simulink model "ECS_FOS"  (Simulink 8.2)
settings: Solver=ode45  StartTime=0.0  StopTime=18000  RelTol=1e-3
InitFcn:
  | load('loss_coeff_mixing_junction.mat')
  | load('SampleOutput.mat')
  | load('HydProp.mat')
  | load('HydraulicLoad.mat')
  | load('initavload.mat')
  | load('SampleFuelBurn.mat')
values from neighbouring files (symbols this model uses):
  FuelBurn = [0 0 0 0 0 0 0 0 0 0 0 0 ... (18249 elements, 1x18249)]    [Benchmark_data1.mat]
  fueltankdata =     [Benchmark_data1.mat]
undefined symbols (not defined in the file or in its folder): AirProp, F1, F2, HUGHES_TREITLER, magnitude, PN_70147, PumpProp
libraries: PowerFlowLib x46, simulink x4
(part 4 of 5)

== system ECS_FOS/ECS/Fuel Tanks/Pumps/Fuel Control Right Wing  ==
  FuelNeed : Inport
  FuelFromPump : Inport  Port=2
  Bus Creator : BusCreator  Inputs=3
  Bus Creator1 : BusCreator  Inputs=3
  Bus Selector : BusSelector  OutputSignals=mdot_kgps,temp_K,pres_kPa
  Gain : Gain
  Gain1 : Gain
  Saturation : Saturate  UpperLimit=inf  LowerLimit=0
  Sum : Sum  Inputs=|+-
  Switch : Switch  Criteria=u2 > Threshold
  Fuel2Engine : Outport
  Fuel2Tank : Outport  Port=2
  wires:
  Gain1/1 -> Bus Creator1/2  "temp_K"
  Gain/1 -> Bus Creator1/3  "pres_kPa"
  Bus Creator1/1 -> Fuel2Engine/1
  Bus Selector/3 -> Gain/1, Bus Creator/3  "<pres_kPa>"
  Switch/1 -> Bus Creator1/1  "mdot_kgps"
  Saturation/1 -> Bus Creator/1  "mdot_kgps"
  Bus Selector/2 -> Gain1/1, Bus Creator/2  "<temp_K>"
  Bus Creator/1 -> Fuel2Tank/1
  Sum/1 -> Switch/2, Saturation/1
  FuelNeed/1 -> Switch/1, Sum/2
  Bus Selector/1 -> Switch/3, Sum/1  "<mdot_kgps>"
  FuelFromPump/1 -> Bus Selector/1

== system ECS_FOS/ECS/Fuel Tanks/Pumps/Fuel Switch On/Off ==
  Right Wing Tank : Inport
  Center Tank : Inport  Port=2
  Left Wing Tank : Inport  Port=3
  Operating RPM : Constant  Value=6000
  Operating RPM1 : Constant  Value=6000
  Operating RPM2 : Constant  Value=6000
  Right Wing Fuel  Pumps On/Off : Switch  Criteria=u2 ~= 0
  Right Wing Fuel  Pumps On/Off1 : Switch  Criteria=u2 ~= 0
  Right Wing Fuel  Pumps On/Off2 : Switch  Criteria=u2 ~= 0
  shut off : Constant  Value=0
  shut off1 : Constant  Value=0
  shut off2 : Constant  Value=0
  Right Wing RPM : Outport
  Left Wing RPM : Outport  Port=2
  Center RPM : Outport  Port=3
  wires:
  Right Wing Fuel  Pumps On/Off2/1 -> Left Wing RPM/1
  Right Wing Fuel  Pumps On/Off1/1 -> Center RPM/1
  Right Wing Fuel  Pumps On/Off/1 -> Right Wing RPM/1
  Left Wing Tank/1 -> Right Wing Fuel  Pumps On/Off2/2
  shut off2/1 -> Right Wing Fuel  Pumps On/Off2/3
  Operating RPM2/1 -> Right Wing Fuel  Pumps On/Off2/1
  Center Tank/1 -> Right Wing Fuel  Pumps On/Off1/2
  shut off1/1 -> Right Wing Fuel  Pumps On/Off1/3
  Operating RPM1/1 -> Right Wing Fuel  Pumps On/Off1/1
  Right Wing Tank/1 -> Right Wing Fuel  Pumps On/Off/2
  shut off/1 -> Right Wing Fuel  Pumps On/Off/3
  Operating RPM/1 -> Right Wing Fuel  Pumps On/Off/1

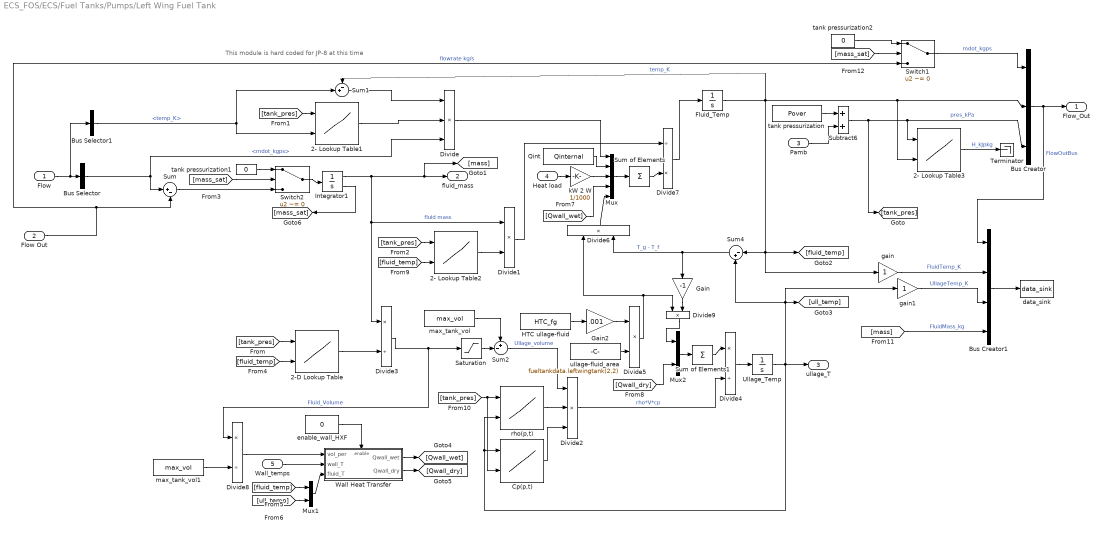
== system ECS_FOS/ECS/Fuel Tanks/Pumps/Left Wing Fuel Tank ==
  note: This module is hard coded for JP-8 at this time
  Flow : Inport
  Flow Out : Inport  Port=2
  Pamb : Inport  Port=3
  Heat load : Inport  Port=4
  Wall_temps : Inport  Port=5
  2- Lookup Table1 : Lookup_n-D  BreakpointsForDimension1=F1.P  BreakpointsForDimension2=F1.T  Table=F1.Cp_pt  RndMeth=Simplest  InputSameDT=on
  2- Lookup Table2 : Lookup_n-D  BreakpointsForDimension1=F1.P  BreakpointsForDimension2=F1.T  Table=F1.Cp_pt  RndMeth=Simplest  InputSameDT=on
  2- Lookup Table3 : Lookup_n-D  BreakpointsForDimension1=F1.P  BreakpointsForDimension2=F1.T  Table=F1.H_pt  RndMeth=Simplest  InputSameDT=on
  2-D Lookup Table : Lookup_n-D  BreakpointsForDimension1=F1.P  BreakpointsForDimension2=F1.T  Table=F1.Rho_pt  RndMeth=Simplest  InputSameDT=on
  Bus Creator : BusCreator  Inputs=3
  Bus Creator1 : BusCreator
  Bus Selector : BusSelector  OutputSignals=mdot_kgps
  Bus Selector1 : BusSelector  OutputSignals=temp_K
  Cp(p,t) : Lookup_n-D  BreakpointsForDimension1=AirProp.P  BreakpointsForDimension2=AirProp.T  Table=AirProp.Cp_pt  RndMeth=Simplest  InputSameDT=on
  Divide : Product  Inputs=***
  Divide{1,5..6,9} (4 alike) : Product  Inputs=**
  Divide2 : Product  Inputs=***
  Divide3 : Product  Inputs=*/
  Divide4 : Product  Inputs=*/
  Divide7 : Product  Inputs=/*
  Divide8 : Product  Inputs=*/
  Fluid_Temp : Integrator  InitialCondition=fld_Tint + 273.15  LimitOutput=on  UpperSaturationLimit=800  LowerSaturationLimit=eps
  Gain : Gain  Gain=-1
  Gain2 : Gain  Gain=.001
  HTC ullage-fluid : Constant  Value=HTC_fg
  Integrator1 : Integrator  InitialCondition=m_init  LimitOutput=on  LowerSaturationLimit=1  ShowSaturationPort=on
  Mux : Mux  Inputs=5
  Mux1 : Mux  Inputs=2
  Mux2 : Mux  Inputs=2
  Qint : Constant  Value=Qinternal
  Saturation : Saturate  UpperLimit=inf  LowerLimit=eps  ZeroCross=off
  Subtract6 : Sum
  Sum : Sum  Inputs=|+-
  Sum of Elements : Sum  Inputs=+
  Sum of Elements1 : Sum  Inputs=+
  Sum1 : Sum  Inputs=-+|
  Sum2 : Sum  Inputs=+-|
  Sum4 : Sum  Inputs=|-+
  Switch1 : Switch  Criteria=u2 ~= 0  Threshold=-1
  Switch2 : Switch  Criteria=u2 ~= 0  Threshold=-1
  Terminator : Terminator
  Ullage_Temp : Integrator  InitialCondition=ull_Tint + 273.15  LimitOutput=on  LowerSaturationLimit=eps
  Wall Heat Transfer : Subsystem  TreatAsAtomicUnit=on
  data_sink : PowerFlowLib/Support Functions//Tools/data_sink
      link override global_data_goto: GotoTag=gdata_PowerFlowLibEnergyPowerSystemsThermalFuelFuelTank
  enable_wall_HXF : Constant  Value=0
  gain : Gain
  gain1 : Gain
  kW 2 W : Gain  Gain=1/1000
  max_tank_vol : Constant  Value=max_vol
  max_tank_vol1 : Constant  Value=max_vol
  rho(p,t) : Lookup_n-D  BreakpointsForDimension1=AirProp.P  BreakpointsForDimension2=AirProp.T  Table=AirProp.Rho_pt  RndMeth=Simplest  InputSameDT=on
  tank pressurization : Constant  Value=Pover
  tank pressurization1 : Constant  Value=0
  tank pressurization2 : Constant  Value=0
  ullage-fluid_area : Constant  Value=fueltankdata.leftwingtank(2,2)
  Flow_Out : Outport
  fluid_mass : Outport  Port=2
  ullage_T : Outport  Port=3
  wires:
  Switch2/1 -> Integrator1/1
  tank pressurization1/1 -> Switch2/1
  [mass_sat] -> Switch2/2
  Integrator1/2 -> [mass_sat]
  Sum/1 -> Switch2/3
  tank pressurization2/1 -> Switch1/1
  [mass_sat] -> Switch1/2
  [mass] -> Bus Creator1/4  "FluidMass_kg"
  gain1/1 -> Bus Creator1/3  "UllageTemp_K"
  gain/1 -> Bus Creator1/2  "FluidTemp_K"
  Bus Creator1/1 -> data_sink/1
  kW 2 W/1 -> Mux/3
  2- Lookup Table3/1 -> Terminator/1  "H_kJpkg"
  Flow/1 -> Bus Selector/1, Bus Selector1/1
  Bus Selector/1 -> Divide/3, Sum/1  "<mdot_kgps>"
  Flow Out/1 -> Sum/2, Switch1/3  "flowrate kg/s"
  Integrator1/1 -> fluid_mass/1, [mass], Divide3/1, Divide1/1  "fluid mass"
  Bus Selector1/1 -> Sum1/2, 2- Lookup Table1/2  "<temp_K>"
  Sum1/1 -> Divide/1
  2- Lookup Table2/1 -> Divide1/2
  rho(p,t)/1 -> Divide2/2
  Cp(p,t)/1 -> Divide2/3
  Divide3/1 -> Saturation/1, Divide8/1  "Fluid_Volume"
  max_tank_vol/1 -> Sum2/1
  Sum2/1 -> Divide2/1  "Ullage_volume"
  Divide4/1 -> Ullage_Temp/1
  Ullage_Temp/1 -> ullage_T/1, gain1/1, Sum4/2, [ull_temp], rho(p,t)/2, Cp(p,t)/1
  Fluid_Temp/1 -> 2- Lookup Table3/2, Bus Creator/2, Sum1/1, gain/1, Sum4/1, [fluid_temp]  "temp_K"
  HTC ullage-fluid/1 -> Gain2/1
  ullage-fluid_area/1 -> Divide5/2
  Sum4/1 -> Divide6/2, Gain/1  "T_g - T_f"
  Divide1/1 -> Divide7/1
  Divide7/1 -> Fluid_Temp/1
  Divide5/1 -> Divide6/1, Divide9/1
  Pamb/1 -> Subtract6/2
  tank pressurization/1 -> Subtract6/1
  Subtract6/1 -> 2- Lookup Table3/1, Bus Creator/3, [tank_pres]  "pres_kPa"
  Bus Creator/1 -> Bus Creator1/1, Flow_Out/1  "FlowOutBus"
  Saturation/1 -> Sum2/2
  [tank_pres] -> 2-D Lookup Table/1
  2-D Lookup Table/1 -> Divide3/2
  [tank_pres] -> 2- Lookup Table1/1
  2- Lookup Table1/1 -> Divide/2
  [tank_pres] -> 2- Lookup Table2/1
  max_tank_vol1/1 -> Divide8/2
  Switch1/1 -> Bus Creator/1  "mdot_kgps"
  Divide/1 -> Mux/1
  Qint/1 -> Mux/2
  Heat load/1 -> kW 2 W/1
  Sum of Elements/1 -> Divide7/2
  Mux/1 -> Sum of Elements/1
  [fluid_temp] -> 2-D Lookup Table/2
  Divide8/1 -> Wall Heat Transfer/1(vol_per)
  Wall_temps/1 -> Wall Heat Transfer/2(wall_T)
  [fluid_temp] -> Mux1/1
  [ull_temp] -> Mux1/2
  Mux1/1 -> Wall Heat Transfer/3(fluid_T)
  Wall Heat Transfer/1(Qwall_wet) -> [Qwall_wet]
  Wall Heat Transfer/2(Qwall_dry) -> [Qwall_dry]
  Divide6/1 -> Mux/5
  Divide2/1 -> Divide4/2  "rho*V*cp"
  Mux2/1 -> Sum of Elements1/1
  Sum of Elements1/1 -> Divide4/1
  Gain/1 -> Divide9/2
  Divide9/1 -> Mux2/1
  [Qwall_dry] -> Mux2/2
  [Qwall_wet] -> Mux/4
  [fluid_temp] -> 2- Lookup Table2/2
  enable_wall_HXF/1 -> Wall Heat Transfer/Enable
  Gain2/1 -> Divide5/1
  [tank_pres] -> rho(p,t)/1, Cp(p,t)/2

== system ECS_FOS/ECS/Fuel Tanks/Pumps/Pump Split1 ==
  Flow In : Inport
  Bus Creator : BusCreator  Inputs=3
  Bus Selector14 : BusSelector  OutputSignals=temp_K,mdot_kgps,pres_kPa
  Gain : Gain  Gain=0.5
  Flow Out : Outport
  wires:
  Bus Selector14/3 -> Bus Creator/3  "<pres_kPa>"
  Gain/1 -> Bus Creator/2  "mdot_kgps"
  Bus Selector14/1 -> Bus Creator/1  "<temp_K>"
  Bus Creator/1 -> Flow Out/1
  Bus Selector14/2 -> Gain/1  "<mdot_kgps>"
  Flow In/1 -> Bus Selector14/1

== system ECS_FOS/ECS/Fuel Tanks/Pumps/Pump Split2 ==
  Flow In : Inport
  Bus Creator : BusCreator  Inputs=3
  Bus Selector14 : BusSelector  OutputSignals=temp_K,mdot_kgps,pres_kPa
  Gain : Gain  Gain=0.5
  Flow Out : Outport
  wires:
  Flow In/1 -> Bus Selector14/1
  Bus Selector14/2 -> Gain/1  "<mdot_kgps>"
  Bus Creator/1 -> Flow Out/1
  Bus Selector14/1 -> Bus Creator/1  "<temp_K>"
  Gain/1 -> Bus Creator/2  "mdot_kgps"
  Bus Selector14/3 -> Bus Creator/3  "<pres_kPa>"

== system ECS_FOS/ECS/Fuel Tanks/Pumps/Pump Split3 ==
  Flow In : Inport
  Bus Creator : BusCreator  Inputs=3
  Bus Selector14 : BusSelector  OutputSignals=temp_K,mdot_kgps,pres_kPa
  Gain : Gain  Gain=0.5
  Flow Out : Outport
  wires:
  Bus Selector14/3 -> Bus Creator/3  "<pres_kPa>"
  Gain/1 -> Bus Creator/2  "mdot_kgps"
  Bus Selector14/1 -> Bus Creator/1  "<temp_K>"
  Bus Creator/1 -> Flow Out/1
  Bus Selector14/2 -> Gain/1  "<mdot_kgps>"
  Flow In/1 -> Bus Selector14/1

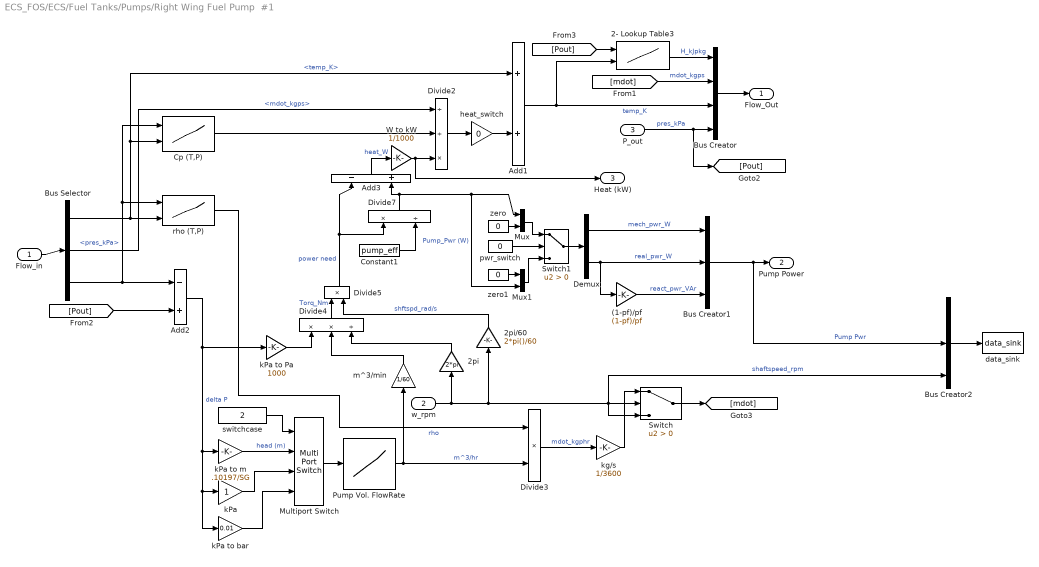
== system ECS_FOS/ECS/Fuel Tanks/Pumps/Right Wing Fuel Pump  #1 ==
  Flow_in : Inport
  w_rpm : Inport  Port=2
  P_out : Inport  Port=3
  (1-pf)/pf : Gain  Gain=(1-pf)/pf
  2- Lookup Table3 : Lookup_n-D  BreakpointsForDimension1=F1.P  BreakpointsForDimension2=F1.T  Table=F1.H_pt  RndMeth=Simplest  InputSameDT=on
  2pi : Gain  Gain=2*pi
  2pi/60 : Gain  Gain=2*pi()/60
  Add1 : Sum
  Add2 : Sum  Inputs=-+
  Add3 : Sum  Inputs=-+
  Bus Creator : BusCreator
  Bus Creator1 : BusCreator  Inputs=3
  Bus Creator2 : BusCreator  Inputs=3
  Bus Selector : BusSelector  OutputSignals=temp_K,mdot_kgps,pres_kPa
  Constant1 : Constant  Value=pump_eff
  Cp (T,P) : Lookup_n-D  BreakpointsForDimension1=F1.P  BreakpointsForDimension2=F1.T  Table=F1.Cp_pt  RndMeth=Simplest  InputSameDT=on
  Demux : Demux  Outputs=2
  Divide2 : Product  Inputs=//*
  Divide3 : Product  Inputs=**
  Divide4 : Product  Inputs=**/
  Divide5 : Product  Inputs=**
  Divide7 : Product  Inputs=*/
  Multiport Switch : MultiPortSwitch
  Mux : Mux  Inputs=2
  Mux1 : Mux  Inputs=2
  Pump Vol. FlowRate : Lookup_n-D  NumberOfTableDimensions=1  BreakpointsForDimension1=PumpProp.B737_AC_fuel1.pres  Table=PumpProp.B737_AC_fuel1.q  RndMeth=Simplest  InputSameDT=on
  Switch : Switch  Criteria=u2 > Threshold
  Switch1 : Switch  Criteria=u2 > Threshold
  W to kW : Gain  Gain=1/1000
  data_sink : PowerFlowLib/Support Functions//Tools/data_sink
  heat_switch : Gain  Gain=0
  "kPa " : Gain
  kPa to Pa : Gain  Gain=1000
  kPa to bar : Gain  Gain=0.01
  kPa to m : Gain  Gain=.10197/SG
  kg/s : Gain  Gain=1/3600
  m^3/min : Gain  Gain=1/60
  pwr_switch : Constant  Value=0
  rho (T,P) : Lookup_n-D  BreakpointsForDimension1=F1.P  BreakpointsForDimension2=F1.T  Table=F1.Rho_pt  RndMeth=Simplest  InputSameDT=on
  switchcase : Constant  Value=2
  zero : Constant  Value=0
  zero1 : Constant  Value=0
  Flow_Out : Outport
  Pump Power : Outport  Port=2
  Heat (kW) : Outport  Port=3
  wires:
  Bus Creator2/1 -> data_sink/1
  heat_switch/1 -> Add1/2
  Mux1/1 -> Switch1/3
  zero1/1 -> Mux1/1
  W to kW/1 -> Divide2/3, Heat (kW)/1
  zero/1 -> Mux/2
  Mux/1 -> Switch1/1
  pwr_switch/1 -> Switch1/2
  Switch1/1 -> Demux/1
  (1-pf)/pf/1 -> Bus Creator1/3  "react_pwr_VAr"
  Demux/2 -> (1-pf)/pf/1, Bus Creator1/2  "real_pwr_W"
  Bus Creator1/1 -> Bus Creator2/2, Pump Power/1  "Pump Pwr"
  Demux/1 -> Bus Creator1/1  "mech_pwr_W"
  Add3/1 -> W to kW/1  "heat_W"
  2pi/1 -> Divide4/3
  Divide7/1 -> Mux1/2, Mux/1, Add3/2  "Pump_Pwr (W)"
  m^3/min/1 -> Divide4/2
  kPa to Pa/1 -> Divide4/1
  Divide5/1 -> Add3/1, Divide7/1  "power need"
  2pi/60/1 -> Divide5/2  "shftspd_rad/s"
  Switch/1 -> [mdot]
  kg/s/1 -> Switch/1
  [Pout] -> 2- Lookup Table3/1
  P_out/1 -> Bus Creator/4, [Pout]  "pres_kPa"
  2- Lookup Table3/1 -> Bus Creator/1  "H_kJpkg"
  Flow_in/1 -> Bus Selector/1
  Bus Creator/1 -> Flow_Out/1
  Divide2/1 -> heat_switch/1
  Cp (T,P)/1 -> Divide2/2
  Constant1/1 -> Divide7/2
  Bus Selector/2 -> Divide2/1  "<mdot_kgps>"
  rho (T,P)/1 -> Divide3/1  "rho"
  Bus Selector/1 -> rho (T,P)/2, Add1/1, Cp (T,P)/2  "<temp_K>"
  Bus Selector/3 -> rho (T,P)/1, Cp (T,P)/1, Add2/1  "<pres_kPa>"
  Add2/1 -> kPa to Pa/1, kPa to m/1, "kPa "/1, kPa to bar/1  "delta P"
  Add1/1 -> 2- Lookup Table3/2, Bus Creator/3  "temp_K"
  w_rpm/1 -> Bus Creator2/3, Switch/3, Switch/2, 2pi/60/1, 2pi/1  "shaftspeed_rpm"
  [mdot] -> Bus Creator/2  "mdot_kgps"
  [Pout] -> Add2/2
  kPa to m/1 -> Multiport Switch/2  "head (m)"
  Divide3/1 -> kg/s/1  "mdot_kgphr"
  Pump Vol. FlowRate/1 -> Divide3/2, m^3/min/1  "m^3/hr"
  Divide4/1 -> Divide5/1  "Torq_Nm"
  switchcase/1 -> Multiport Switch/1
  Multiport Switch/1 -> Pump Vol. FlowRate/1
  "kPa "/1 -> Multiport Switch/3
  kPa to bar/1 -> Multiport Switch/4

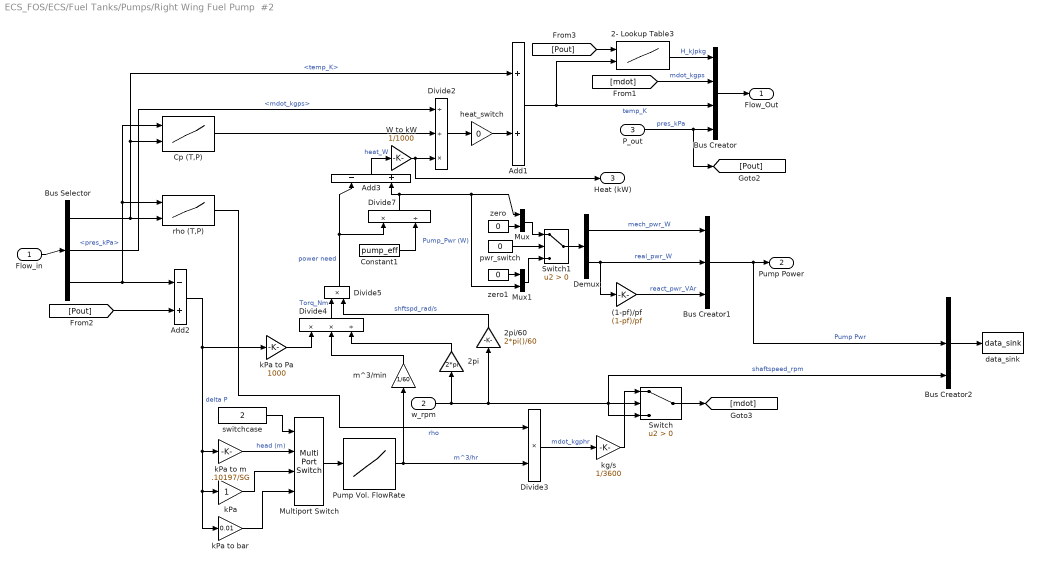
== system ECS_FOS/ECS/Fuel Tanks/Pumps/Right Wing Fuel Pump  #2 ==
  Flow_in : Inport
  w_rpm : Inport  Port=2
  P_out : Inport  Port=3
  (1-pf)/pf : Gain  Gain=(1-pf)/pf
  2- Lookup Table3 : Lookup_n-D  BreakpointsForDimension1=F1.P  BreakpointsForDimension2=F1.T  Table=F1.H_pt  RndMeth=Simplest  InputSameDT=on
  2pi : Gain  Gain=2*pi
  2pi/60 : Gain  Gain=2*pi()/60
  Add1 : Sum
  Add2 : Sum  Inputs=-+
  Add3 : Sum  Inputs=-+
  Bus Creator : BusCreator
  Bus Creator1 : BusCreator  Inputs=3
  Bus Creator2 : BusCreator  Inputs=3
  Bus Selector : BusSelector  OutputSignals=temp_K,mdot_kgps,pres_kPa
  Constant1 : Constant  Value=pump_eff
  Cp (T,P) : Lookup_n-D  BreakpointsForDimension1=F1.P  BreakpointsForDimension2=F1.T  Table=F1.Cp_pt  RndMeth=Simplest  InputSameDT=on
  Demux : Demux  Outputs=2
  Divide2 : Product  Inputs=//*
  Divide3 : Product  Inputs=**
  Divide4 : Product  Inputs=**/
  Divide5 : Product  Inputs=**
  Divide7 : Product  Inputs=*/
  Multiport Switch : MultiPortSwitch
  Mux : Mux  Inputs=2
  Mux1 : Mux  Inputs=2
  Pump Vol. FlowRate : Lookup_n-D  NumberOfTableDimensions=1  BreakpointsForDimension1=PumpProp.B737_AC_fuel1.pres  Table=PumpProp.B737_AC_fuel1.q  RndMeth=Simplest  InputSameDT=on
  Switch : Switch  Criteria=u2 > Threshold
  Switch1 : Switch  Criteria=u2 > Threshold
  W to kW : Gain  Gain=1/1000
  data_sink : PowerFlowLib/Support Functions//Tools/data_sink
  heat_switch : Gain  Gain=0
  "kPa " : Gain
  kPa to Pa : Gain  Gain=1000
  kPa to bar : Gain  Gain=0.01
  kPa to m : Gain  Gain=.10197/SG
  kg/s : Gain  Gain=1/3600
  m^3/min : Gain  Gain=1/60
  pwr_switch : Constant  Value=0
  rho (T,P) : Lookup_n-D  BreakpointsForDimension1=F1.P  BreakpointsForDimension2=F1.T  Table=F1.Rho_pt  RndMeth=Simplest  InputSameDT=on
  switchcase : Constant  Value=2
  zero : Constant  Value=0
  zero1 : Constant  Value=0
  Flow_Out : Outport
  Pump Power : Outport  Port=2
  Heat (kW) : Outport  Port=3
  wires:
  kPa to bar/1 -> Multiport Switch/4
  "kPa "/1 -> Multiport Switch/3
  Multiport Switch/1 -> Pump Vol. FlowRate/1
  switchcase/1 -> Multiport Switch/1
  Divide4/1 -> Divide5/1  "Torq_Nm"
  Pump Vol. FlowRate/1 -> m^3/min/1, Divide3/2  "m^3/hr"
  Divide3/1 -> kg/s/1  "mdot_kgphr"
  kPa to m/1 -> Multiport Switch/2  "head (m)"
  [Pout] -> Add2/2
  [mdot] -> Bus Creator/2  "mdot_kgps"
  w_rpm/1 -> 2pi/1, 2pi/60/1, Switch/2, Switch/3, Bus Creator2/3  "shaftspeed_rpm"
  Add1/1 -> Bus Creator/3, 2- Lookup Table3/2  "temp_K"
  Add2/1 -> kPa to bar/1, "kPa "/1, kPa to m/1, kPa to Pa/1  "delta P"
  Bus Selector/3 -> Add2/1, Cp (T,P)/1, rho (T,P)/1  "<pres_kPa>"
  Bus Selector/1 -> Cp (T,P)/2, Add1/1, rho (T,P)/2  "<temp_K>"
  rho (T,P)/1 -> Divide3/1  "rho"
  Bus Selector/2 -> Divide2/1  "<mdot_kgps>"
  Constant1/1 -> Divide7/2
  Cp (T,P)/1 -> Divide2/2
  Divide2/1 -> heat_switch/1
  Bus Creator/1 -> Flow_Out/1
  Flow_in/1 -> Bus Selector/1
  2- Lookup Table3/1 -> Bus Creator/1  "H_kJpkg"
  P_out/1 -> [Pout], Bus Creator/4  "pres_kPa"
  [Pout] -> 2- Lookup Table3/1
  kg/s/1 -> Switch/1
  Switch/1 -> [mdot]
  2pi/60/1 -> Divide5/2  "shftspd_rad/s"
  Divide5/1 -> Divide7/1, Add3/1  "power need"
  kPa to Pa/1 -> Divide4/1
  m^3/min/1 -> Divide4/2
  Divide7/1 -> Add3/2, Mux/1, Mux1/2  "Pump_Pwr (W)"
  2pi/1 -> Divide4/3
  Add3/1 -> W to kW/1  "heat_W"
  Demux/1 -> Bus Creator1/1  "mech_pwr_W"
  Bus Creator1/1 -> Pump Power/1, Bus Creator2/2  "Pump Pwr"
  Demux/2 -> Bus Creator1/2, (1-pf)/pf/1  "real_pwr_W"
  (1-pf)/pf/1 -> Bus Creator1/3  "react_pwr_VAr"
  Switch1/1 -> Demux/1
  pwr_switch/1 -> Switch1/2
  Mux/1 -> Switch1/1
  zero/1 -> Mux/2
  W to kW/1 -> Heat (kW)/1, Divide2/3
  zero1/1 -> Mux1/1
  Mux1/1 -> Switch1/3
  heat_switch/1 -> Add1/2
  Bus Creator2/1 -> data_sink/1

== system ECS_FOS/ECS/Fuel Tanks/Pumps/Right Wing Fuel Pump  #3 ==
  Flow_in : Inport
  w_rpm : Inport  Port=2
  P_out : Inport  Port=3
  (1-pf)/pf : Gain  Gain=(1-pf)/pf
  2- Lookup Table3 : Lookup_n-D  BreakpointsForDimension1=F1.P  BreakpointsForDimension2=F1.T  Table=F1.H_pt  RndMeth=Simplest  InputSameDT=on
  2pi : Gain  Gain=2*pi
  2pi/60 : Gain  Gain=2*pi()/60
  Add1 : Sum
  Add2 : Sum  Inputs=-+
  Add3 : Sum  Inputs=-+
  Bus Creator : BusCreator
  Bus Creator1 : BusCreator  Inputs=3
  Bus Creator2 : BusCreator  Inputs=3
  Bus Selector : BusSelector  OutputSignals=temp_K,mdot_kgps,pres_kPa
  Constant1 : Constant  Value=pump_eff
  Cp (T,P) : Lookup_n-D  BreakpointsForDimension1=F1.P  BreakpointsForDimension2=F1.T  Table=F1.Cp_pt  RndMeth=Simplest  InputSameDT=on
  Demux : Demux  Outputs=2
  Divide2 : Product  Inputs=//*
  Divide3 : Product  Inputs=**
  Divide4 : Product  Inputs=**/
  Divide5 : Product  Inputs=**
  Divide7 : Product  Inputs=*/
  Multiport Switch : MultiPortSwitch
  Mux : Mux  Inputs=2
  Mux1 : Mux  Inputs=2
  Pump Vol. FlowRate : Lookup_n-D  NumberOfTableDimensions=1  BreakpointsForDimension1=PumpProp.B737_AC_fuel1.pres  Table=PumpProp.B737_AC_fuel1.q  RndMeth=Simplest  InputSameDT=on
  Switch : Switch  Criteria=u2 > Threshold
  Switch1 : Switch  Criteria=u2 > Threshold
  W to kW : Gain  Gain=1/1000
  data_sink : PowerFlowLib/Support Functions//Tools/data_sink
  heat_switch : Gain  Gain=0
  "kPa " : Gain
  kPa to Pa : Gain  Gain=1000
  kPa to bar : Gain  Gain=0.01
  kPa to m : Gain  Gain=.10197/SG
  kg/s : Gain  Gain=1/3600
  m^3/min : Gain  Gain=1/60
  pwr_switch : Constant  Value=0
  rho (T,P) : Lookup_n-D  BreakpointsForDimension1=F1.P  BreakpointsForDimension2=F1.T  Table=F1.Rho_pt  RndMeth=Simplest  InputSameDT=on
  switchcase : Constant  Value=2
  zero : Constant  Value=0
  zero1 : Constant  Value=0
  Flow_Out : Outport
  Pump Power : Outport  Port=2
  Heat (kW) : Outport  Port=3
  wires:
  Bus Creator2/1 -> data_sink/1
  heat_switch/1 -> Add1/2
  Mux1/1 -> Switch1/3
  zero1/1 -> Mux1/1
  W to kW/1 -> Divide2/3, Heat (kW)/1
  zero/1 -> Mux/2
  Mux/1 -> Switch1/1
  pwr_switch/1 -> Switch1/2
  Switch1/1 -> Demux/1
  (1-pf)/pf/1 -> Bus Creator1/3  "react_pwr_VAr"
  Demux/2 -> (1-pf)/pf/1, Bus Creator1/2  "real_pwr_W"
  Bus Creator1/1 -> Bus Creator2/2, Pump Power/1  "Pump Pwr"
  Demux/1 -> Bus Creator1/1  "mech_pwr_W"
  Add3/1 -> W to kW/1  "heat_W"
  2pi/1 -> Divide4/3
  Divide7/1 -> Mux1/2, Mux/1, Add3/2  "Pump_Pwr (W)"
  m^3/min/1 -> Divide4/2
  kPa to Pa/1 -> Divide4/1
  Divide5/1 -> Add3/1, Divide7/1  "power need"
  2pi/60/1 -> Divide5/2  "shftspd_rad/s"
  Switch/1 -> [mdot]
  kg/s/1 -> Switch/1
  [Pout] -> 2- Lookup Table3/1
  P_out/1 -> Bus Creator/4, [Pout]  "pres_kPa"
  2- Lookup Table3/1 -> Bus Creator/1  "H_kJpkg"
  Flow_in/1 -> Bus Selector/1
  Bus Creator/1 -> Flow_Out/1
  Divide2/1 -> heat_switch/1
  Cp (T,P)/1 -> Divide2/2
  Constant1/1 -> Divide7/2
  Bus Selector/2 -> Divide2/1  "<mdot_kgps>"
  rho (T,P)/1 -> Divide3/1  "rho"
  Bus Selector/1 -> rho (T,P)/2, Add1/1, Cp (T,P)/2  "<temp_K>"
  Bus Selector/3 -> rho (T,P)/1, Cp (T,P)/1, Add2/1  "<pres_kPa>"
  Add2/1 -> kPa to Pa/1, kPa to m/1, "kPa "/1, kPa to bar/1  "delta P"
  Add1/1 -> 2- Lookup Table3/2, Bus Creator/3  "temp_K"
  w_rpm/1 -> Bus Creator2/3, Switch/3, Switch/2, 2pi/60/1, 2pi/1  "shaftspeed_rpm"
  [mdot] -> Bus Creator/2  "mdot_kgps"
  [Pout] -> Add2/2
  kPa to m/1 -> Multiport Switch/2  "head (m)"
  Divide3/1 -> kg/s/1  "mdot_kgphr"
  Pump Vol. FlowRate/1 -> Divide3/2, m^3/min/1  "m^3/hr"
  Divide4/1 -> Divide5/1  "Torq_Nm"
  switchcase/1 -> Multiport Switch/1
  Multiport Switch/1 -> Pump Vol. FlowRate/1
  "kPa "/1 -> Multiport Switch/3
  kPa to bar/1 -> Multiport Switch/4

== system ECS_FOS/ECS/Fuel Tanks/Pumps/Right Wing Fuel Pump  #4 ==
  Flow_in : Inport
  w_rpm : Inport  Port=2
  P_out : Inport  Port=3
  (1-pf)/pf : Gain  Gain=(1-pf)/pf
  2- Lookup Table3 : Lookup_n-D  BreakpointsForDimension1=F1.P  BreakpointsForDimension2=F1.T  Table=F1.H_pt  RndMeth=Simplest  InputSameDT=on
  2pi : Gain  Gain=2*pi
  2pi/60 : Gain  Gain=2*pi()/60
  Add1 : Sum
  Add2 : Sum  Inputs=-+
  Add3 : Sum  Inputs=-+
  Bus Creator : BusCreator
  Bus Creator1 : BusCreator  Inputs=3
  Bus Creator2 : BusCreator  Inputs=3
  Bus Selector : BusSelector  OutputSignals=temp_K,mdot_kgps,pres_kPa
  Constant1 : Constant  Value=pump_eff
  Cp (T,P) : Lookup_n-D  BreakpointsForDimension1=F1.P  BreakpointsForDimension2=F1.T  Table=F1.Cp_pt  RndMeth=Simplest  InputSameDT=on
  Demux : Demux  Outputs=2
  Divide2 : Product  Inputs=//*
  Divide3 : Product  Inputs=**
  Divide4 : Product  Inputs=**/
  Divide5 : Product  Inputs=**
  Divide7 : Product  Inputs=*/
  Multiport Switch : MultiPortSwitch
  Mux : Mux  Inputs=2
  Mux1 : Mux  Inputs=2
  Pump Vol. FlowRate : Lookup_n-D  NumberOfTableDimensions=1  BreakpointsForDimension1=PumpProp.B737_AC_fuel1.pres  Table=PumpProp.B737_AC_fuel1.q  RndMeth=Simplest  InputSameDT=on
  Switch : Switch  Criteria=u2 > Threshold
  Switch1 : Switch  Criteria=u2 > Threshold
  W to kW : Gain  Gain=1/1000
  data_sink : PowerFlowLib/Support Functions//Tools/data_sink
  heat_switch : Gain  Gain=0
  "kPa " : Gain
  kPa to Pa : Gain  Gain=1000
  kPa to bar : Gain  Gain=0.01
  kPa to m : Gain  Gain=.10197/SG
  kg/s : Gain  Gain=1/3600
  m^3/min : Gain  Gain=1/60
  pwr_switch : Constant  Value=0
  rho (T,P) : Lookup_n-D  BreakpointsForDimension1=F1.P  BreakpointsForDimension2=F1.T  Table=F1.Rho_pt  RndMeth=Simplest  InputSameDT=on
  switchcase : Constant  Value=2
  zero : Constant  Value=0
  zero1 : Constant  Value=0
  Flow_Out : Outport
  Pump Power : Outport  Port=2
  Heat (kW) : Outport  Port=3
  wires:
  kPa to bar/1 -> Multiport Switch/4
  "kPa "/1 -> Multiport Switch/3
  Multiport Switch/1 -> Pump Vol. FlowRate/1
  switchcase/1 -> Multiport Switch/1
  Divide4/1 -> Divide5/1  "Torq_Nm"
  Pump Vol. FlowRate/1 -> m^3/min/1, Divide3/2  "m^3/hr"
  Divide3/1 -> kg/s/1  "mdot_kgphr"
  kPa to m/1 -> Multiport Switch/2  "head (m)"
  [Pout] -> Add2/2
  [mdot] -> Bus Creator/2  "mdot_kgps"
  w_rpm/1 -> 2pi/1, 2pi/60/1, Switch/2, Switch/3, Bus Creator2/3  "shaftspeed_rpm"
  Add1/1 -> Bus Creator/3, 2- Lookup Table3/2  "temp_K"
  Add2/1 -> kPa to bar/1, "kPa "/1, kPa to m/1, kPa to Pa/1  "delta P"
  Bus Selector/3 -> Add2/1, Cp (T,P)/1, rho (T,P)/1  "<pres_kPa>"
  Bus Selector/1 -> Cp (T,P)/2, Add1/1, rho (T,P)/2  "<temp_K>"
  rho (T,P)/1 -> Divide3/1  "rho"
  Bus Selector/2 -> Divide2/1  "<mdot_kgps>"
  Constant1/1 -> Divide7/2
  Cp (T,P)/1 -> Divide2/2
  Divide2/1 -> heat_switch/1
  Bus Creator/1 -> Flow_Out/1
  Flow_in/1 -> Bus Selector/1
  2- Lookup Table3/1 -> Bus Creator/1  "H_kJpkg"
  P_out/1 -> [Pout], Bus Creator/4  "pres_kPa"
  [Pout] -> 2- Lookup Table3/1
  kg/s/1 -> Switch/1
  Switch/1 -> [mdot]
  2pi/60/1 -> Divide5/2  "shftspd_rad/s"
  Divide5/1 -> Divide7/1, Add3/1  "power need"
  kPa to Pa/1 -> Divide4/1
  m^3/min/1 -> Divide4/2
  Divide7/1 -> Add3/2, Mux/1, Mux1/2  "Pump_Pwr (W)"
  2pi/1 -> Divide4/3
  Add3/1 -> W to kW/1  "heat_W"
  Demux/1 -> Bus Creator1/1  "mech_pwr_W"
  Bus Creator1/1 -> Pump Power/1, Bus Creator2/2  "Pump Pwr"
  Demux/2 -> Bus Creator1/2, (1-pf)/pf/1  "real_pwr_W"
  (1-pf)/pf/1 -> Bus Creator1/3  "react_pwr_VAr"
  Switch1/1 -> Demux/1
  pwr_switch/1 -> Switch1/2
  Mux/1 -> Switch1/1
  zero/1 -> Mux/2
  W to kW/1 -> Heat (kW)/1, Divide2/3
  zero1/1 -> Mux1/1
  Mux1/1 -> Switch1/3
  heat_switch/1 -> Add1/2
  Bus Creator2/1 -> data_sink/1

== system ECS_FOS/ECS/Fuel Tanks/Pumps/Right Wing Fuel Pump  #5 ==
  Flow_in : Inport
  w_rpm : Inport  Port=2
  P_out : Inport  Port=3
  (1-pf)/pf : Gain  Gain=(1-pf)/pf
  2- Lookup Table3 : Lookup_n-D  BreakpointsForDimension1=F1.P  BreakpointsForDimension2=F1.T  Table=F1.H_pt  RndMeth=Simplest  InputSameDT=on
  2pi : Gain  Gain=2*pi
  2pi/60 : Gain  Gain=2*pi()/60
  Add1 : Sum
  Add2 : Sum  Inputs=-+
  Add3 : Sum  Inputs=-+
  Bus Creator : BusCreator
  Bus Creator1 : BusCreator  Inputs=3
  Bus Creator2 : BusCreator  Inputs=3
  Bus Selector : BusSelector  OutputSignals=temp_K,mdot_kgps,pres_kPa
  Constant1 : Constant  Value=pump_eff
  Cp (T,P) : Lookup_n-D  BreakpointsForDimension1=F1.P  BreakpointsForDimension2=F1.T  Table=F1.Cp_pt  RndMeth=Simplest  InputSameDT=on
  Demux : Demux  Outputs=2
  Divide2 : Product  Inputs=//*
  Divide3 : Product  Inputs=**
  Divide4 : Product  Inputs=**/
  Divide5 : Product  Inputs=**
  Divide7 : Product  Inputs=*/
  Multiport Switch : MultiPortSwitch
  Mux : Mux  Inputs=2
  Mux1 : Mux  Inputs=2
  Pump Vol. FlowRate : Lookup_n-D  NumberOfTableDimensions=1  BreakpointsForDimension1=PumpProp.B737_AC_fuel1.pres  Table=PumpProp.B737_AC_fuel1.q  RndMeth=Simplest  InputSameDT=on
  Switch : Switch  Criteria=u2 > Threshold
  Switch1 : Switch  Criteria=u2 > Threshold
  W to kW : Gain  Gain=1/1000
  data_sink : PowerFlowLib/Support Functions//Tools/data_sink
  heat_switch : Gain  Gain=0
  "kPa " : Gain
  kPa to Pa : Gain  Gain=1000
  kPa to bar : Gain  Gain=0.01
  kPa to m : Gain  Gain=.10197/SG
  kg/s : Gain  Gain=1/3600
  m^3/min : Gain  Gain=1/60
  pwr_switch : Constant  Value=0
  rho (T,P) : Lookup_n-D  BreakpointsForDimension1=F1.P  BreakpointsForDimension2=F1.T  Table=F1.Rho_pt  RndMeth=Simplest  InputSameDT=on
  switchcase : Constant  Value=2
  zero : Constant  Value=0
  zero1 : Constant  Value=0
  Flow_Out : Outport
  Pump Power : Outport  Port=2
  Heat (kW) : Outport  Port=3
  wires:
  Bus Creator2/1 -> data_sink/1
  heat_switch/1 -> Add1/2
  Mux1/1 -> Switch1/3
  zero1/1 -> Mux1/1
  W to kW/1 -> Divide2/3, Heat (kW)/1
  zero/1 -> Mux/2
  Mux/1 -> Switch1/1
  pwr_switch/1 -> Switch1/2
  Switch1/1 -> Demux/1
  (1-pf)/pf/1 -> Bus Creator1/3  "react_pwr_VAr"
  Demux/2 -> (1-pf)/pf/1, Bus Creator1/2  "real_pwr_W"
  Bus Creator1/1 -> Bus Creator2/2, Pump Power/1  "Pump Pwr"
  Demux/1 -> Bus Creator1/1  "mech_pwr_W"
  Add3/1 -> W to kW/1  "heat_W"
  2pi/1 -> Divide4/3
  Divide7/1 -> Mux1/2, Mux/1, Add3/2  "Pump_Pwr (W)"
  m^3/min/1 -> Divide4/2
  kPa to Pa/1 -> Divide4/1
  Divide5/1 -> Add3/1, Divide7/1  "power need"
  2pi/60/1 -> Divide5/2  "shftspd_rad/s"
  Switch/1 -> [mdot]
  kg/s/1 -> Switch/1
  [Pout] -> 2- Lookup Table3/1
  P_out/1 -> Bus Creator/4, [Pout]  "pres_kPa"
  2- Lookup Table3/1 -> Bus Creator/1  "H_kJpkg"
  Flow_in/1 -> Bus Selector/1
  Bus Creator/1 -> Flow_Out/1
  Divide2/1 -> heat_switch/1
  Cp (T,P)/1 -> Divide2/2
  Constant1/1 -> Divide7/2
  Bus Selector/2 -> Divide2/1  "<mdot_kgps>"
  rho (T,P)/1 -> Divide3/1  "rho"
  Bus Selector/1 -> rho (T,P)/2, Add1/1, Cp (T,P)/2  "<temp_K>"
  Bus Selector/3 -> rho (T,P)/1, Cp (T,P)/1, Add2/1  "<pres_kPa>"
  Add2/1 -> kPa to Pa/1, kPa to m/1, "kPa "/1, kPa to bar/1  "delta P"
  Add1/1 -> 2- Lookup Table3/2, Bus Creator/3  "temp_K"
  w_rpm/1 -> Bus Creator2/3, Switch/3, Switch/2, 2pi/60/1, 2pi/1  "shaftspeed_rpm"
  [mdot] -> Bus Creator/2  "mdot_kgps"
  [Pout] -> Add2/2
  kPa to m/1 -> Multiport Switch/2  "head (m)"
  Divide3/1 -> kg/s/1  "mdot_kgphr"
  Pump Vol. FlowRate/1 -> Divide3/2, m^3/min/1  "m^3/hr"
  Divide4/1 -> Divide5/1  "Torq_Nm"
  switchcase/1 -> Multiport Switch/1
  Multiport Switch/1 -> Pump Vol. FlowRate/1
  "kPa "/1 -> Multiport Switch/3
  kPa to bar/1 -> Multiport Switch/4

== system ECS_FOS/ECS/Fuel Tanks/Pumps/Right Wing Fuel Pump  #6 ==
  Flow_in : Inport
  w_rpm : Inport  Port=2
  P_out : Inport  Port=3
  (1-pf)/pf : Gain  Gain=(1-pf)/pf
  2- Lookup Table3 : Lookup_n-D  BreakpointsForDimension1=F1.P  BreakpointsForDimension2=F1.T  Table=F1.H_pt  RndMeth=Simplest  InputSameDT=on
  2pi : Gain  Gain=2*pi
  2pi/60 : Gain  Gain=2*pi()/60
  Add1 : Sum
  Add2 : Sum  Inputs=-+
  Add3 : Sum  Inputs=-+
  Bus Creator : BusCreator
  Bus Creator1 : BusCreator  Inputs=3
  Bus Creator2 : BusCreator  Inputs=3
  Bus Selector : BusSelector  OutputSignals=temp_K,mdot_kgps,pres_kPa
  Constant1 : Constant  Value=pump_eff
  Cp (T,P) : Lookup_n-D  BreakpointsForDimension1=F1.P  BreakpointsForDimension2=F1.T  Table=F1.Cp_pt  RndMeth=Simplest  InputSameDT=on
  Demux : Demux  Outputs=2
  Divide2 : Product  Inputs=//*
  Divide3 : Product  Inputs=**
  Divide4 : Product  Inputs=**/
  Divide5 : Product  Inputs=**
  Divide7 : Product  Inputs=*/
  Multiport Switch : MultiPortSwitch
  Mux : Mux  Inputs=2
  Mux1 : Mux  Inputs=2
  Pump Vol. FlowRate : Lookup_n-D  NumberOfTableDimensions=1  BreakpointsForDimension1=PumpProp.B737_AC_fuel1.pres  Table=PumpProp.B737_AC_fuel1.q  RndMeth=Simplest  InputSameDT=on
  Switch : Switch  Criteria=u2 > Threshold
  Switch1 : Switch  Criteria=u2 > Threshold
  W to kW : Gain  Gain=1/1000
  data_sink : PowerFlowLib/Support Functions//Tools/data_sink
  heat_switch : Gain  Gain=0
  "kPa " : Gain
  kPa to Pa : Gain  Gain=1000
  kPa to bar : Gain  Gain=0.01
  kPa to m : Gain  Gain=.10197/SG
  kg/s : Gain  Gain=1/3600
  m^3/min : Gain  Gain=1/60
  pwr_switch : Constant  Value=0
  rho (T,P) : Lookup_n-D  BreakpointsForDimension1=F1.P  BreakpointsForDimension2=F1.T  Table=F1.Rho_pt  RndMeth=Simplest  InputSameDT=on
  switchcase : Constant  Value=2
  zero : Constant  Value=0
  zero1 : Constant  Value=0
  Flow_Out : Outport
  Pump Power : Outport  Port=2
  Heat (kW) : Outport  Port=3
  wires:
  kPa to bar/1 -> Multiport Switch/4
  "kPa "/1 -> Multiport Switch/3
  Multiport Switch/1 -> Pump Vol. FlowRate/1
  switchcase/1 -> Multiport Switch/1
  Divide4/1 -> Divide5/1  "Torq_Nm"
  Pump Vol. FlowRate/1 -> m^3/min/1, Divide3/2  "m^3/hr"
  Divide3/1 -> kg/s/1  "mdot_kgphr"
  kPa to m/1 -> Multiport Switch/2  "head (m)"
  [Pout] -> Add2/2
  [mdot] -> Bus Creator/2  "mdot_kgps"
  w_rpm/1 -> 2pi/1, 2pi/60/1, Switch/2, Switch/3, Bus Creator2/3  "shaftspeed_rpm"
  Add1/1 -> Bus Creator/3, 2- Lookup Table3/2  "temp_K"
  Add2/1 -> kPa to bar/1, "kPa "/1, kPa to m/1, kPa to Pa/1  "delta P"
  Bus Selector/3 -> Add2/1, Cp (T,P)/1, rho (T,P)/1  "<pres_kPa>"
  Bus Selector/1 -> Cp (T,P)/2, Add1/1, rho (T,P)/2  "<temp_K>"
  rho (T,P)/1 -> Divide3/1  "rho"
  Bus Selector/2 -> Divide2/1  "<mdot_kgps>"
  Constant1/1 -> Divide7/2
  Cp (T,P)/1 -> Divide2/2
  Divide2/1 -> heat_switch/1
  Bus Creator/1 -> Flow_Out/1
  Flow_in/1 -> Bus Selector/1
  2- Lookup Table3/1 -> Bus Creator/1  "H_kJpkg"
  P_out/1 -> [Pout], Bus Creator/4  "pres_kPa"
  [Pout] -> 2- Lookup Table3/1
  kg/s/1 -> Switch/1
  Switch/1 -> [mdot]
  2pi/60/1 -> Divide5/2  "shftspd_rad/s"
  Divide5/1 -> Divide7/1, Add3/1  "power need"
  kPa to Pa/1 -> Divide4/1
  m^3/min/1 -> Divide4/2
  Divide7/1 -> Add3/2, Mux/1, Mux1/2  "Pump_Pwr (W)"
  2pi/1 -> Divide4/3
  Add3/1 -> W to kW/1  "heat_W"
  Demux/1 -> Bus Creator1/1  "mech_pwr_W"
  Bus Creator1/1 -> Pump Power/1, Bus Creator2/2  "Pump Pwr"
  Demux/2 -> Bus Creator1/2, (1-pf)/pf/1  "real_pwr_W"
  (1-pf)/pf/1 -> Bus Creator1/3  "react_pwr_VAr"
  Switch1/1 -> Demux/1
  pwr_switch/1 -> Switch1/2
  Mux/1 -> Switch1/1
  zero/1 -> Mux/2
  W to kW/1 -> Heat (kW)/1, Divide2/3
  zero1/1 -> Mux1/1
  Mux1/1 -> Switch1/3
  heat_switch/1 -> Add1/2
  Bus Creator2/1 -> data_sink/1

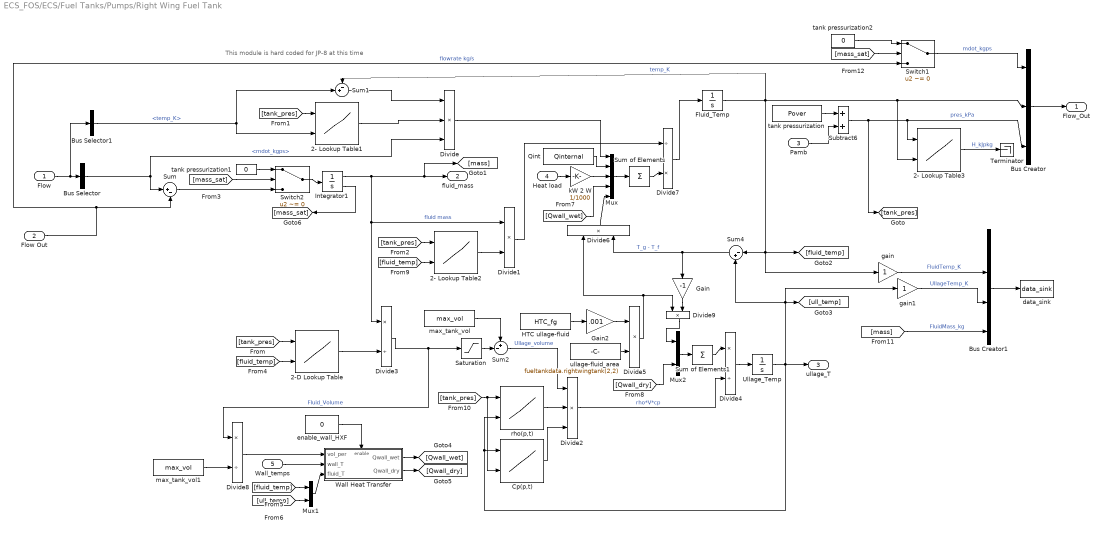
== system ECS_FOS/ECS/Fuel Tanks/Pumps/Right Wing Fuel Tank ==
  note: This module is hard coded for JP-8 at this time
  Flow : Inport
  Flow Out : Inport  Port=2
  Pamb : Inport  Port=3
  Heat load : Inport  Port=4
  Wall_temps : Inport  Port=5
  2- Lookup Table1 : Lookup_n-D  BreakpointsForDimension1=F1.P  BreakpointsForDimension2=F1.T  Table=F1.Cp_pt  RndMeth=Simplest  InputSameDT=on
  2- Lookup Table2 : Lookup_n-D  BreakpointsForDimension1=F1.P  BreakpointsForDimension2=F1.T  Table=F1.Cp_pt  RndMeth=Simplest  InputSameDT=on
  2- Lookup Table3 : Lookup_n-D  BreakpointsForDimension1=F1.P  BreakpointsForDimension2=F1.T  Table=F1.H_pt  RndMeth=Simplest  InputSameDT=on
  2-D Lookup Table : Lookup_n-D  BreakpointsForDimension1=F1.P  BreakpointsForDimension2=F1.T  Table=F1.Rho_pt  RndMeth=Simplest  InputSameDT=on
  Bus Creator : BusCreator  Inputs=3
  Bus Creator1 : BusCreator
  Bus Selector : BusSelector  OutputSignals=mdot_kgps
  Bus Selector1 : BusSelector  OutputSignals=temp_K
  Cp(p,t) : Lookup_n-D  BreakpointsForDimension1=AirProp.P  BreakpointsForDimension2=AirProp.T  Table=AirProp.Cp_pt  RndMeth=Simplest  InputSameDT=on
  Divide : Product  Inputs=***
  Divide{1,5..6,9} (4 alike) : Product  Inputs=**
  Divide2 : Product  Inputs=***
  Divide3 : Product  Inputs=*/
  Divide4 : Product  Inputs=*/
  Divide7 : Product  Inputs=/*
  Divide8 : Product  Inputs=*/
  Fluid_Temp : Integrator  InitialCondition=fld_Tint + 273.15  LimitOutput=on  UpperSaturationLimit=800  LowerSaturationLimit=eps
  Gain : Gain  Gain=-1
  Gain2 : Gain  Gain=.001
  HTC ullage-fluid : Constant  Value=HTC_fg
  Integrator1 : Integrator  InitialCondition=m_init  LimitOutput=on  LowerSaturationLimit=1  ShowSaturationPort=on
  Mux : Mux  Inputs=5
  Mux1 : Mux  Inputs=2
  Mux2 : Mux  Inputs=2
  Qint : Constant  Value=Qinternal
  Saturation : Saturate  UpperLimit=inf  LowerLimit=eps  ZeroCross=off
  Subtract6 : Sum
  Sum : Sum  Inputs=|+-
  Sum of Elements : Sum  Inputs=+
  Sum of Elements1 : Sum  Inputs=+
  Sum1 : Sum  Inputs=-+|
  Sum2 : Sum  Inputs=+-|
  Sum4 : Sum  Inputs=|-+
  Switch1 : Switch  Criteria=u2 ~= 0  Threshold=-1
  Switch2 : Switch  Criteria=u2 ~= 0  Threshold=-1
  Terminator : Terminator
  Ullage_Temp : Integrator  InitialCondition=ull_Tint + 273.15  LimitOutput=on  LowerSaturationLimit=eps
  Wall Heat Transfer : Subsystem  TreatAsAtomicUnit=on
  data_sink : PowerFlowLib/Support Functions//Tools/data_sink
      link override global_data_goto: GotoTag=gdata_PowerFlowLibEnergyPowerSystemsThermalFuelFuelTank
  enable_wall_HXF : Constant  Value=0
  gain : Gain
  gain1 : Gain
  kW 2 W : Gain  Gain=1/1000
  max_tank_vol : Constant  Value=max_vol
  max_tank_vol1 : Constant  Value=max_vol
  rho(p,t) : Lookup_n-D  BreakpointsForDimension1=AirProp.P  BreakpointsForDimension2=AirProp.T  Table=AirProp.Rho_pt  RndMeth=Simplest  InputSameDT=on
  tank pressurization : Constant  Value=Pover
  tank pressurization1 : Constant  Value=0
  tank pressurization2 : Constant  Value=0
  ullage-fluid_area : Constant  Value=fueltankdata.rightwingtank(2,2)
  Flow_Out : Outport
  fluid_mass : Outport  Port=2
  ullage_T : Outport  Port=3
  wires:
  Switch2/1 -> Integrator1/1
  tank pressurization1/1 -> Switch2/1
  [mass_sat] -> Switch2/2
  Integrator1/2 -> [mass_sat]
  Sum/1 -> Switch2/3
  tank pressurization2/1 -> Switch1/1
  [mass_sat] -> Switch1/2
  [mass] -> Bus Creator1/4  "FluidMass_kg"
  gain1/1 -> Bus Creator1/3  "UllageTemp_K"
  gain/1 -> Bus Creator1/2  "FluidTemp_K"
  Bus Creator1/1 -> data_sink/1
  kW 2 W/1 -> Mux/3
  2- Lookup Table3/1 -> Terminator/1  "H_kJpkg"
  Flow/1 -> Bus Selector/1, Bus Selector1/1
  Bus Selector/1 -> Divide/3, Sum/1  "<mdot_kgps>"
  Flow Out/1 -> Sum/2, Switch1/3  "flowrate kg/s"
  Integrator1/1 -> fluid_mass/1, [mass], Divide3/1, Divide1/1  "fluid mass"
  Bus Selector1/1 -> Sum1/2, 2- Lookup Table1/2  "<temp_K>"
  Sum1/1 -> Divide/1
  2- Lookup Table2/1 -> Divide1/2
  rho(p,t)/1 -> Divide2/2
  Cp(p,t)/1 -> Divide2/3
  Divide3/1 -> Saturation/1, Divide8/1  "Fluid_Volume"
  max_tank_vol/1 -> Sum2/1
  Sum2/1 -> Divide2/1  "Ullage_volume"
  Divide4/1 -> Ullage_Temp/1
  Ullage_Temp/1 -> ullage_T/1, gain1/1, Sum4/2, [ull_temp], rho(p,t)/2, Cp(p,t)/1
  Fluid_Temp/1 -> 2- Lookup Table3/2, Bus Creator/2, Sum1/1, gain/1, Sum4/1, [fluid_temp]  "temp_K"
  HTC ullage-fluid/1 -> Gain2/1
  ullage-fluid_area/1 -> Divide5/2
  Sum4/1 -> Divide6/2, Gain/1  "T_g - T_f"
  Divide1/1 -> Divide7/1
  Divide7/1 -> Fluid_Temp/1
  Divide5/1 -> Divide6/1, Divide9/1
  Pamb/1 -> Subtract6/2
  tank pressurization/1 -> Subtract6/1
  Subtract6/1 -> 2- Lookup Table3/1, Bus Creator/3, [tank_pres]  "pres_kPa"
  Bus Creator/1 -> Flow_Out/1
  Saturation/1 -> Sum2/2
  [tank_pres] -> 2-D Lookup Table/1
  2-D Lookup Table/1 -> Divide3/2
  [tank_pres] -> 2- Lookup Table1/1
  2- Lookup Table1/1 -> Divide/2
  [tank_pres] -> 2- Lookup Table2/1
  max_tank_vol1/1 -> Divide8/2
  Switch1/1 -> Bus Creator/1  "mdot_kgps"
  Divide/1 -> Mux/1
  Qint/1 -> Mux/2
  Heat load/1 -> kW 2 W/1
  Sum of Elements/1 -> Divide7/2
  Mux/1 -> Sum of Elements/1
  [fluid_temp] -> 2-D Lookup Table/2
  Divide8/1 -> Wall Heat Transfer/1(vol_per)
  Wall_temps/1 -> Wall Heat Transfer/2(wall_T)
  [fluid_temp] -> Mux1/1
  [ull_temp] -> Mux1/2
  Mux1/1 -> Wall Heat Transfer/3(fluid_T)
  Wall Heat Transfer/1(Qwall_wet) -> [Qwall_wet]
  Wall Heat Transfer/2(Qwall_dry) -> [Qwall_dry]
  Divide6/1 -> Mux/5
  Divide2/1 -> Divide4/2  "rho*V*cp"
  Mux2/1 -> Sum of Elements1/1
  Sum of Elements1/1 -> Divide4/1
  Gain/1 -> Divide9/2
  Divide9/1 -> Mux2/1
  [Qwall_dry] -> Mux2/2
  [Qwall_wet] -> Mux/4
  [fluid_temp] -> 2- Lookup Table2/2
  enable_wall_HXF/1 -> Wall Heat Transfer/Enable
  Gain2/1 -> Divide5/1
  [tank_pres] -> rho(p,t)/1, Cp(p,t)/2

== system ECS_FOS/ECS/Left PACK/Distribution of bleed air ==
  Bleed to Valve : Inport
  Bleed to ACM : Inport  Port=2
  bleed_temp : Inport  Port=3
  bleed_pres : Inport  Port=4
  Bus Creator1 : BusCreator  Inputs=3
  Bus Creator2 : BusCreator  Inputs=3
  Scope : Scope  NumInputPorts=4
      settings: YMin=0~386.7~110~0.2  YMax=0.055~387.8~160~0.85  SaveName=ScopeData42  SampleInput=on  SampleTime=1
  Flow to Mix Junc. : Outport
  Flow to HX : Outport  Port=2
  wires:
  Bus Creator2/1 -> Flow to HX/1
  Bus Creator1/1 -> Flow to Mix Junc./1
  Bleed to Valve/1 -> Scope/1, Bus Creator1/1  "mdot_kgps"
  bleed_pres/1 -> Scope/3, Bus Creator1/3, Bus Creator2/3
  bleed_temp/1 -> Scope/2, Bus Creator1/2, Bus Creator2/2
  Bleed to ACM/1 -> Scope/4, Bus Creator2/1  "mdot_kgps"

== system ECS_FOS/ECS/Left PACK/Ram air inlet ==
  Temp_amb : Inport
  Temp_comp : Inport  Port=2
  2 : Constant  Value=T_35
  Bus Creator : BusCreator  Inputs=3
  Bus Selector4 : BusSelector  OutputSignals=temp_K
  Constant1 : Constant  Value=22.5
  Gain : Gain  Gain=0.95
  Gain1 : Gain
  Memory : Memory  X0=ram_air
  Subtract : Sum  Inputs=+-
  Switch : Switch  Criteria=u2 ~= 0  Threshold=30
  Flow Out : Outport
  wires:
  Gain1/1 -> Switch/1
  Memory/1 -> Gain/1, Gain1/1, Bus Creator/3  "mdot_kgps"
  Bus Creator/1 -> Flow Out/1
  Constant1/1 -> Bus Creator/2  "pres_kPa"
  Temp_amb/1 -> Bus Creator/1  "temp_K"
  Switch/1 -> Memory/1
  Gain/1 -> Switch/3
  Subtract/1 -> Switch/2
  2/1 -> Subtract/2
  Bus Selector4/1 -> Subtract/1  "<temp_K>"
  Temp_comp/1 -> Bus Selector4/1

== system ECS_FOS/ECS/Left PACK/Subsystem1 ==
  Bypass Ratio : Inport
  Air from PHX : Inport  Port=2
  Bus Creator : BusCreator  Inputs=3
  Bus Creator1 : BusCreator  Inputs=3
  Bus Selector : BusSelector  OutputSignals=mdot_kgps,temp_K,pres_kPa
  Fcn1 : Fcn  Expr=1-u(1)
  Gain : Gain
  Gain1 : Gain
  Gain2 : Gain
  Product : Product  RndMeth=Zero
  Product1 : Product  RndMeth=Zero
  Saturation : Saturate  UpperLimit=inf  LowerLimit=eps
  Air to Mix Junc : Outport
  Air to Comp : Outport  Port=2
  wires:
  Gain2/1 -> Bus Creator/3  "pres_kPa"
  Fcn1/1 -> Product/1
  Bypass Ratio/1 -> Product1/2, Fcn1/1
  Product/1 -> Saturation/1
  Air from PHX/1 -> Bus Selector/1
  Bus Selector/1 -> Product1/1, Product/2  "<mdot_kgps>"
  Bus Creator/1 -> Air to Comp/1
  Bus Selector/2 -> Bus Creator/2, Gain1/1  "<temp_K>"
  Saturation/1 -> Bus Creator/1  "mdot_kgps"
  Product1/1 -> Bus Creator1/1  "mdot_kgps"
  Bus Selector/3 -> Gain2/1, Gain/1  "<pres_kPa>"
  Bus Creator1/1 -> Air to Mix Junc/1
  Gain/1 -> Bus Creator1/3  "pres_kPa"
  Gain1/1 -> Bus Creator1/2  "temp_K"

== system ECS_FOS/ECS/Left PACK/User-set_ supply_pressure ==
  Flow In : Inport
  Cabin Pres. : Inport  Port=2
  Bus Creator4 : BusCreator  Inputs=3
  Bus Selector3 : BusSelector  OutputSignals=mdot_kgps,temp_K
  Gain1 : Gain  Gain=1.1
  Flow Out : Outport
  wires:
  Cabin Pres./1 -> Gain1/1
  Bus Creator4/1 -> Flow Out/1
  Flow In/1 -> Bus Selector3/1
  Gain1/1 -> Bus Creator4/3  "pres_kPa"
  Bus Selector3/2 -> Bus Creator4/2  "<temp_K>"
  Bus Selector3/1 -> Bus Creator4/1  "<mdot_kgps>"

== system ECS_FOS/ECS/Left PACK/Valve1 ==
  Flow In : Inport
  Bus Creator2 : BusCreator  Inputs=3
  Bus Selector2 : BusSelector  OutputSignals=mdot_kgps,pres_kPa,temp_K
  Math Functin : Math  Operator=pow  SaturateOnIntegerOverflow=on
  Product : Product  RndMeth=Zero
  Sum : Sum  Inputs=|-+
  "Value?? -- MAW" : Constant  Value=50
  get u : Gain
  mass_flow_rate1 : Constant  Value=2
  Flow Out : Outport
  wires:
  "Value?? -- MAW"/1 -> Product/1
  Bus Selector2/3 -> Bus Creator2/3  "<temp_K>"
  Sum/1 -> Bus Creator2/2  "pres_kPa"
  Bus Selector2/2 -> Sum/2  "<pres_kPa>"
  Product/1 -> Sum/1
  Math Functin/1 -> Product/2
  mass_flow_rate1/1 -> Math Functin/2
  get u/1 -> Math Functin/1
  Bus Selector2/1 -> get u/1, Bus Creator2/1  "<mdot_kgps>"
  Flow In/1 -> Bus Selector2/1
  Bus Creator2/1 -> Flow Out/1

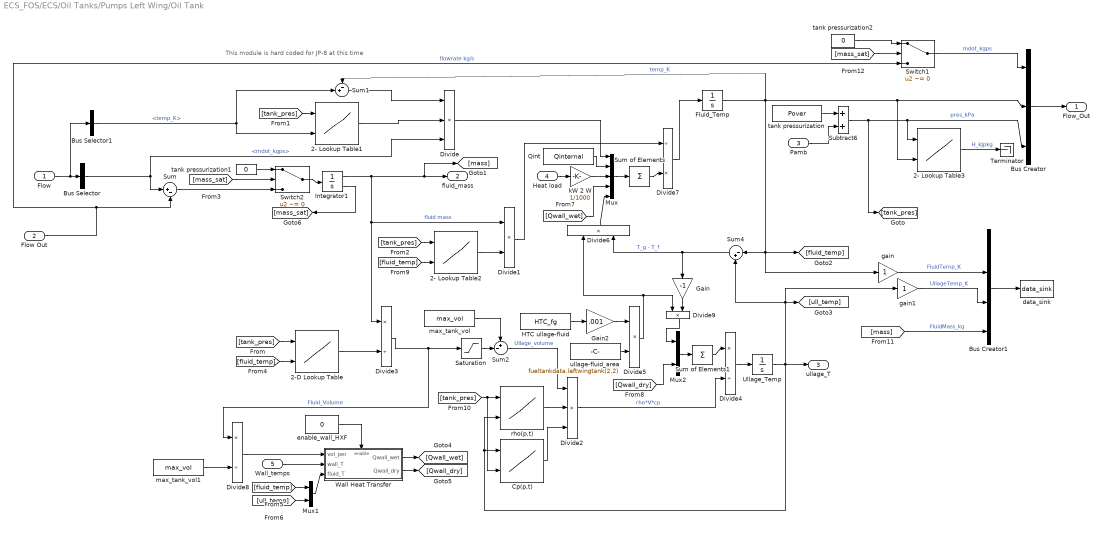
== system ECS_FOS/ECS/Oil Tanks/Pumps Left Wing/Oil Tank ==
  note: This module is hard coded for JP-8 at this time
  Flow : Inport
  Flow Out : Inport  Port=2
  Pamb : Inport  Port=3
  Heat load : Inport  Port=4
  Wall_temps : Inport  Port=5
  2- Lookup Table1 : Lookup_n-D  BreakpointsForDimension1=F1.P  BreakpointsForDimension2=F1.T  Table=F1.Cp_pt  RndMeth=Simplest  InputSameDT=on
  2- Lookup Table2 : Lookup_n-D  BreakpointsForDimension1=F1.P  BreakpointsForDimension2=F1.T  Table=F1.Cp_pt  RndMeth=Simplest  InputSameDT=on
  2- Lookup Table3 : Lookup_n-D  BreakpointsForDimension1=F1.P  BreakpointsForDimension2=F1.T  Table=F1.H_pt  RndMeth=Simplest  InputSameDT=on
  2-D Lookup Table : Lookup_n-D  BreakpointsForDimension1=F1.P  BreakpointsForDimension2=F1.T  Table=F1.Rho_pt  RndMeth=Simplest  InputSameDT=on
  Bus Creator : BusCreator  Inputs=3
  Bus Creator1 : BusCreator
  Bus Selector : BusSelector  OutputSignals=mdot_kgps
  Bus Selector1 : BusSelector  OutputSignals=temp_K
  Cp(p,t) : Lookup_n-D  BreakpointsForDimension1=AirProp.P  BreakpointsForDimension2=AirProp.T  Table=AirProp.Cp_pt  RndMeth=Simplest  InputSameDT=on
  Divide : Product  Inputs=***
  Divide{1,5..6,9} (4 alike) : Product  Inputs=**
  Divide2 : Product  Inputs=***
  Divide3 : Product  Inputs=*/
  Divide4 : Product  Inputs=*/
  Divide7 : Product  Inputs=/*
  Divide8 : Product  Inputs=*/
  Fluid_Temp : Integrator  InitialCondition=fld_Tint + 273.15  LimitOutput=on  UpperSaturationLimit=800  LowerSaturationLimit=eps
  Gain : Gain  Gain=-1
  Gain2 : Gain  Gain=.001
  HTC ullage-fluid : Constant  Value=HTC_fg
  Integrator1 : Integrator  InitialCondition=m_init  LimitOutput=on  LowerSaturationLimit=1  ShowSaturationPort=on
  Mux : Mux  Inputs=5
  Mux1 : Mux  Inputs=2
  Mux2 : Mux  Inputs=2
  Qint : Constant  Value=Qinternal
  Saturation : Saturate  UpperLimit=inf  LowerLimit=eps  ZeroCross=off
  Subtract6 : Sum
  Sum : Sum  Inputs=|+-
  Sum of Elements : Sum  Inputs=+
  Sum of Elements1 : Sum  Inputs=+
  Sum1 : Sum  Inputs=-+|
  Sum2 : Sum  Inputs=+-|
  Sum4 : Sum  Inputs=|-+
  Switch1 : Switch  Criteria=u2 ~= 0  Threshold=-1
  Switch2 : Switch  Criteria=u2 ~= 0  Threshold=-1
  Terminator : Terminator
  Ullage_Temp : Integrator  InitialCondition=ull_Tint + 273.15  LimitOutput=on  LowerSaturationLimit=eps
  Wall Heat Transfer : Subsystem  TreatAsAtomicUnit=on
  data_sink : PowerFlowLib/Support Functions//Tools/data_sink
      link override global_data_goto: GotoTag=gdata_PowerFlowLibEnergyPowerSystemsThermalFuelFuelTank
  enable_wall_HXF : Constant  Value=0
  gain : Gain
  gain1 : Gain
  kW 2 W : Gain  Gain=1/1000
  max_tank_vol : Constant  Value=max_vol
  max_tank_vol1 : Constant  Value=max_vol
  rho(p,t) : Lookup_n-D  BreakpointsForDimension1=AirProp.P  BreakpointsForDimension2=AirProp.T  Table=AirProp.Rho_pt  RndMeth=Simplest  InputSameDT=on
  tank pressurization : Constant  Value=Pover
  tank pressurization1 : Constant  Value=0
  tank pressurization2 : Constant  Value=0
  ullage-fluid_area : Constant  Value=fueltankdata.leftwingtank(2,2)
  Flow_Out : Outport
  fluid_mass : Outport  Port=2
  ullage_T : Outport  Port=3
  wires:
  Switch2/1 -> Integrator1/1
  tank pressurization1/1 -> Switch2/1
  [mass_sat] -> Switch2/2
  Integrator1/2 -> [mass_sat]
  Sum/1 -> Switch2/3
  tank pressurization2/1 -> Switch1/1
  [mass_sat] -> Switch1/2
  [mass] -> Bus Creator1/4  "FluidMass_kg"
  gain1/1 -> Bus Creator1/3  "UllageTemp_K"
  gain/1 -> Bus Creator1/2  "FluidTemp_K"
  Bus Creator1/1 -> data_sink/1
  kW 2 W/1 -> Mux/3
  2- Lookup Table3/1 -> Terminator/1  "H_kJpkg"
  Flow/1 -> Bus Selector/1, Bus Selector1/1
  Bus Selector/1 -> Divide/3, Sum/1  "<mdot_kgps>"
  Flow Out/1 -> Sum/2, Switch1/3  "flowrate kg/s"
  Integrator1/1 -> fluid_mass/1, [mass], Divide3/1, Divide1/1  "fluid mass"
  Bus Selector1/1 -> Sum1/2, 2- Lookup Table1/2  "<temp_K>"
  Sum1/1 -> Divide/1
  2- Lookup Table2/1 -> Divide1/2
  rho(p,t)/1 -> Divide2/2
  Cp(p,t)/1 -> Divide2/3
  Divide3/1 -> Saturation/1, Divide8/1  "Fluid_Volume"
  max_tank_vol/1 -> Sum2/1
  Sum2/1 -> Divide2/1  "Ullage_volume"
  Divide4/1 -> Ullage_Temp/1
  Ullage_Temp/1 -> ullage_T/1, gain1/1, Sum4/2, [ull_temp], rho(p,t)/2, Cp(p,t)/1
  Fluid_Temp/1 -> 2- Lookup Table3/2, Bus Creator/2, Sum1/1, gain/1, Sum4/1, [fluid_temp]  "temp_K"
  HTC ullage-fluid/1 -> Gain2/1
  ullage-fluid_area/1 -> Divide5/2
  Sum4/1 -> Divide6/2, Gain/1  "T_g - T_f"
  Divide1/1 -> Divide7/1
  Divide7/1 -> Fluid_Temp/1
  Divide5/1 -> Divide6/1, Divide9/1
  Pamb/1 -> Subtract6/2
  tank pressurization/1 -> Subtract6/1
  Subtract6/1 -> 2- Lookup Table3/1, Bus Creator/3, [tank_pres]  "pres_kPa"
  Bus Creator/1 -> Flow_Out/1
  Saturation/1 -> Sum2/2
  [tank_pres] -> 2-D Lookup Table/1
  2-D Lookup Table/1 -> Divide3/2
  [tank_pres] -> 2- Lookup Table1/1
  2- Lookup Table1/1 -> Divide/2
  [tank_pres] -> 2- Lookup Table2/1
  max_tank_vol1/1 -> Divide8/2
  Switch1/1 -> Bus Creator/1  "mdot_kgps"
  Divide/1 -> Mux/1
  Qint/1 -> Mux/2
  Heat load/1 -> kW 2 W/1
  Sum of Elements/1 -> Divide7/2
  Mux/1 -> Sum of Elements/1
  [fluid_temp] -> 2-D Lookup Table/2
  Divide8/1 -> Wall Heat Transfer/1(vol_per)
  Wall_temps/1 -> Wall Heat Transfer/2(wall_T)
  [fluid_temp] -> Mux1/1
  [ull_temp] -> Mux1/2
  Mux1/1 -> Wall Heat Transfer/3(fluid_T)
  Wall Heat Transfer/1(Qwall_wet) -> [Qwall_wet]
  Wall Heat Transfer/2(Qwall_dry) -> [Qwall_dry]
  Divide6/1 -> Mux/5
  Divide2/1 -> Divide4/2  "rho*V*cp"
  Mux2/1 -> Sum of Elements1/1
  Sum of Elements1/1 -> Divide4/1
  Gain/1 -> Divide9/2
  Divide9/1 -> Mux2/1
  [Qwall_dry] -> Mux2/2
  [Qwall_wet] -> Mux/4
  [fluid_temp] -> 2- Lookup Table2/2
  enable_wall_HXF/1 -> Wall Heat Transfer/Enable
  Gain2/1 -> Divide5/1
  [tank_pres] -> rho(p,t)/1, Cp(p,t)/2
